simulink model "PID_Control"  (R2024b)
settings: Solver=VariableStepAuto  StartTime=0.0  StopTime=10.0  RelTol=1e-3
settings Model: Creator=nroberts  LastModifiedBy=nroberts
settings SolverCC: DateTimeAtSimulationTimeZero=[]

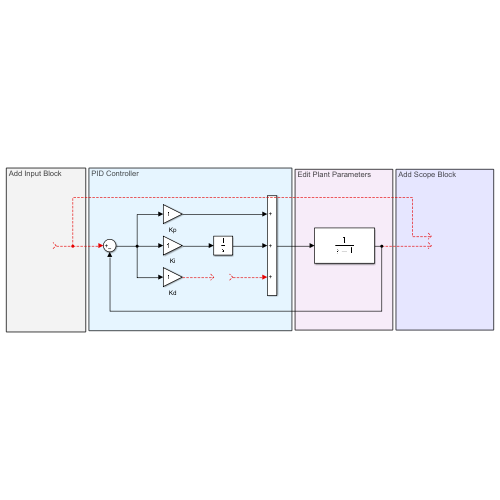
[thumbnail: Simulink's stored preview of the top-level diagram]
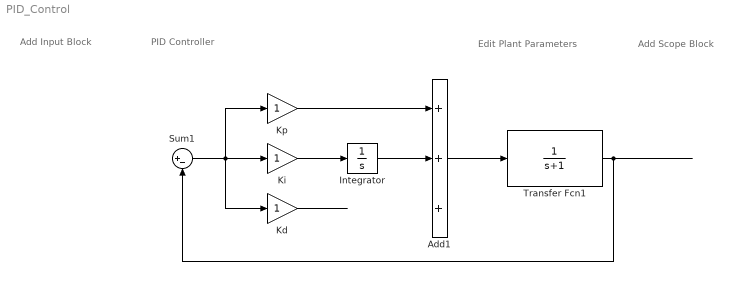
== system PID_Control ==
  note: Edit Plant Parameters
  note: PID Controller
  note: Add Input Block
  note: Add Scope Block
  Add1 : Sum  Inputs=+++
  Integrator : Integrator
  Kd : Gain
  Ki : Gain
  Kp : Gain
  Sum1 : Sum  Inputs=|+-
  Transfer Fcn1 : TransferFcn  Denominator=[1 1]
  wires:
  Add1/1 -> Transfer Fcn1/1
  Transfer Fcn1/1 -> Sum1/2
  ? -> Add1/3
  Kd/1 -> ?
  Sum1/1 -> Kp/1, Kd/1, Ki/1
  Integrator/1 -> Add1/2
  Ki/1 -> Integrator/1
  ? -> Sum1/1
  Kp/1 -> Add1/1
